simulink model "hearingAid_System_v1"  (R2026a)
settings: Solver=VariableStepAuto
undefined symbols (not defined in the file): bHigh, bLow, bMid, dspblkCoreblockFVToolHelper, gcbh
libraries: audiodynamicrange x2, dspstat3 x2, dspmathops x2, audiofilters x2, dspvision x1, dspsnks4 x1, dspsigops x1
settings Model: Creator=admin  LastModifiedBy=shami

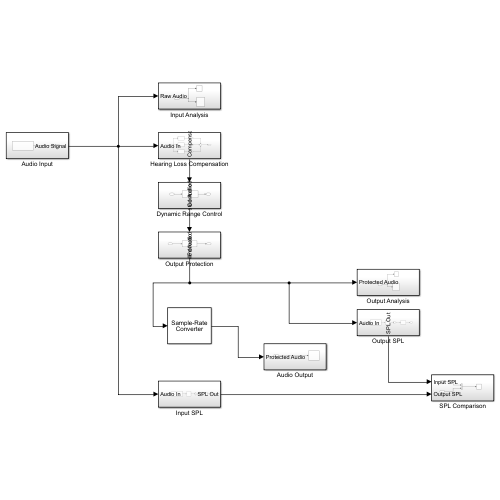
[thumbnail: Simulink's stored preview of the top-level diagram]
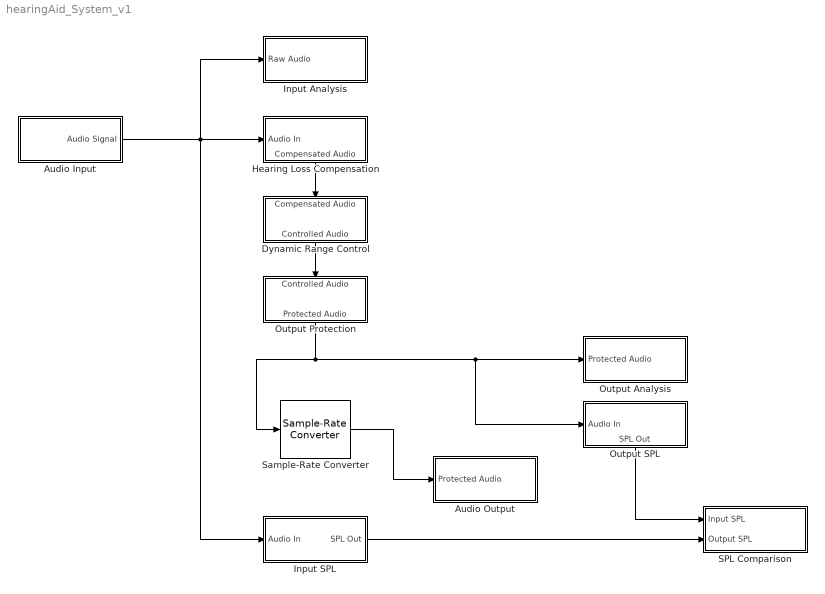
== system hearingAid_System_v1 ==
  Audio Input : Subsystem
  Audio Output : Subsystem
  Dynamic Range Control : Subsystem  Description=|
      | Controls the amplitude dynamics of the compensated signal using compression followed by 
      | peak limiting. The compressor reduces excessive level variations, while the limiter prevents 
      | high-amplitude transients from exceeding the selected threshold.
      settings: PortSchema="{\"entries\":[{\"content\":{\"sides\":[{\"content\":{},\"type\":\"ConnectorPlacement.EquallySpacedRectSide\",\"uuid\":\"9fa1bc4c-7734-4da4-8790-dcaf3a5a96d7\"},{\"content\":{\"side\":\"RIGHT\"},\"type\":\"ConnectorPlacement.EquallySpacedRectSide\",\"uuid\":\"a0bb4f64-da4e-44f2-8384-5606d89d98dc\"},{\"content\":{\"connectorIds\":[\"In1\"],\"side\":\"TOP\"},\"type\":\"ConnectorPlacement.EquallySpacedRectSide\",\"uuid\":\"07e91a7b-911d-4066-a5e2-6f66f183605b\"},{\"content\":{\"connectorIds\":[\"Out1\"],\"side\":\"BOTTOM\"},\"type\":\"ConnectorPlacement.EquallySpacedRectSide\",\"uuid\":\"dc75b34e-663d-4060-af1f-fa3536e55f2f\"}]},\"type\":\"ConnectorPlacement.EquallySpacedConnector\",\"uuid\":\"5366c7c7-2506-4129-8805-fe24e186531d\"}],\"packageUris\":[\"http://schema.mathworks.com/mf0/Connector/R2020b\"],\"version\":\"1.0\"}"
  Hearing Loss Compensation : Subsystem  Description=|
      | Separates the input audio into low-, mid-, and high-frequency bands using matched-delay 
      | FIR filters. Independent prescription gains are applied to each band and the signals are 
      | recombined to produce the compensated audio signal.
      settings: PortSchema="{\"entries\":[{\"content\":{\"sides\":[{\"content\":{\"connectorIds\":[\"In1\"]},\"type\":\"ConnectorPlacement.EquallySpacedRectSide\",\"uuid\":\"9fa1bc4c-7734-4da4-8790-dcaf3a5a96d7\"},{\"content\":{\"side\":\"RIGHT\"},\"type\":\"ConnectorPlacement.EquallySpacedRectSide\",\"uuid\":\"a0bb4f64-da4e-44f2-8384-5606d89d98dc\"},{\"content\":{\"side\":\"TOP\"},\"type\":\"ConnectorPlacement.EquallySpacedRectSide\",\"uuid\":\"07e91a7b-911d-4066-a5e2-6f66f183605b\"},{\"content\":{\"connectorIds\":[\"Out1\"],\"side\":\"BOTTOM\"},\"type\":\"ConnectorPlacement.EquallySpacedRectSide\",\"uuid\":\"08ca0ef5-9875-4344-8c5b-4fbce4711590\"}]},\"type\":\"ConnectorPlacement.EquallySpacedConnector\",\"uuid\":\"5366c7c7-2506-4129-8805-fe24e186531d\"}],\"packageUris\":[\"http://schema.mathworks.com/mf0/Connector/R2020b\"],\"version\":\"1.0\"}"
  Input Analysis : Subsystem  Description=|
      | Analyzes the incoming audio signal in the time and frequency domains before hearing-aid 
      | processing. The subsystem provides waveform and spectral views of the original signal for 
      | comparison with the processed output.
  Input SPL : Subsystem  Description=|
      | Estimates the A-weighted sound pressure level of the input audio using frequency weighting 
      | and moving RMS measurement. The resulting level is provided for real-time monitoring and 
      | comparison with the processed signal.
  Output Analysis : Subsystem  Description=|
      | Monitors the processed audio in the time and frequency domains after dynamic range control. 
      | The waveform and spectrum provide direct evidence of changes introduced by the hearing-aid 
      | processing chain.
  Output Protection : Subsystem  Description=|
      | Protects the compensated audio from excessive amplitude peaks before playback. The 
      | subsystem applies final peak-level control to prevent clipping and maintain a controlled 
      | signal level for the downstream audio output stage.
      settings: PortSchema="{\"entries\":[{\"content\":{\"sides\":[{\"content\":{},\"type\":\"ConnectorPlacement.EquallySpacedRectSide\",\"uuid\":\"9fa1bc4c-7734-4da4-8790-dcaf3a5a96d7\"},{\"content\":{\"side\":\"RIGHT\"},\"type\":\"ConnectorPlacement.EquallySpacedRectSide\",\"uuid\":\"a0bb4f64-da4e-44f2-8384-5606d89d98dc\"},{\"content\":{\"connectorIds\":[\"In1\"],\"side\":\"TOP\"},\"type\":\"ConnectorPlacement.EquallySpacedRectSide\",\"uuid\":\"07e91a7b-911d-4066-a5e2-6f66f183605b\"},{\"content\":{\"connectorIds\":[\"Out1\"],\"side\":\"BOTTOM\"},\"type\":\"ConnectorPlacement.EquallySpacedRectSide\",\"uuid\":\"e48d2dd4-e7e7-47b9-be68-aa31b977a762\"}]},\"type\":\"ConnectorPlacement.EquallySpacedConnector\",\"uuid\":\"5366c7c7-2506-4129-8805-fe24e186531d\"}],\"packageUris\":[\"http://schema.mathworks.com/mf0/Connector/R2020b\"],\"version\":\"1.0\"}"
  Output SPL : Subsystem  Description=|
      | Measures the A-weighted sound pressure level after hearing-aid processing using the same 
      | measurement chain as the input stage, enabling a consistent input-versus-output level 
      | comparison.
      settings: PortSchema="{\"entries\":[{\"content\":{\"sides\":[{\"content\":{\"connectorIds\":[\"In1\"]},\"type\":\"ConnectorPlacement.EquallySpacedRectSide\",\"uuid\":\"9fa1bc4c-7734-4da4-8790-dcaf3a5a96d7\"},{\"content\":{\"side\":\"RIGHT\"},\"type\":\"ConnectorPlacement.EquallySpacedRectSide\",\"uuid\":\"a0bb4f64-da4e-44f2-8384-5606d89d98dc\"},{\"content\":{\"side\":\"TOP\"},\"type\":\"ConnectorPlacement.EquallySpacedRectSide\",\"uuid\":\"07e91a7b-911d-4066-a5e2-6f66f183605b\"},{\"content\":{\"connectorIds\":[\"Out1\"],\"side\":\"BOTTOM\"},\"type\":\"ConnectorPlacement.EquallySpacedRectSide\",\"uuid\":\"6873dc33-1ba5-4860-bfcc-e1687ab0e849\"}]},\"type\":\"ConnectorPlacement.EquallySpacedConnector\",\"uuid\":\"5366c7c7-2506-4129-8805-fe24e186531d\"}],\"packageUris\":[\"http://schema.mathworks.com/mf0/Connector/R2020b\"],\"version\":\"1.0\"}"
  SPL Comparison : Subsystem  Description=|
      | Compares the measured input and output sound pressure levels on a common time axis to 
      | visualize the level changes produced by the hearing-aid processing system.
  Sample-Rate Converter : dspsigops/Sample-Rate Converter  InputSampleRate=16000  OutputSampleRate=48000  OutputRateTolerance=0  Bandwidth=7500  StopbandAttenuation=80  AllowArbitraryInputLength=off  SimulateUsing=Interpreted execution
      settings: LibrarySourceBlock=|
      | dspmlti4/Sample-Rate
      | Converter
  wires:
  Sample-Rate Converter/1 -> Audio Output/1(Protected Audio)
  Dynamic Range Control/1(Controlled Audio) -> Output Protection/1(Controlled Audio)
  Output SPL/1(SPL Out) -> SPL Comparison/1(Input SPL)
  Hearing Loss Compensation/1(Compensated Audio) -> Dynamic Range Control/1(Compensated Audio)
  Audio Input/1(Audio Signal) -> Input SPL/1(Audio In), Input Analysis/1(Raw Audio), Hearing Loss Compensation/1(Audio In)
  Output Protection/1(Protected Audio) -> Output Analysis/1(Protected Audio), Output SPL/1(Audio In), Sample-Rate Converter/1
  Input SPL/1(SPL Out) -> SPL Comparison/2(Output SPL)

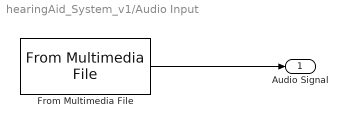
== system hearingAid_System_v1/Audio Input ==
  From Multimedia File : dspvision/From Multimedia File  inputFilename=E:\SS Project\Simulink-Hearing-Aid\Data\datasets\TIMIT\TRAIN\DR1\FCJF0\SA1.WAV  readRange=[1 Inf]  loop=on  numPlays=1  outputStreams=Audio only  videoDataType=single  audioDataType=double  inheritSampleTime=on  userDefinedSampleTime=1/30  noAudioOutput=off  isIntensityVideo=off  fourcc=RGB  colorVideoFormat=Separate color signals  outputEOF=off  dataOrg=Column-major  audioFrameSize=1024  computeAudioFrameSize=off  outSamplingMode=Sample based
      settings: LibrarySourceBlock=audiosources/From Multimedia File
  Audio Signal : Outport
  wires:
  From Multimedia File/1 -> Audio Signal/1

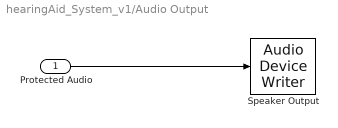
== system hearingAid_System_v1/Audio Output ==
  Protected Audio : Inport
  Speaker Output : dspsnks4/Audio Device Writer  Driver=DirectSound  Device=Default  InheritSampleRate=off  SampleRate=44100  BitDepth=16-bit integer  BufferSize=4096  NumBuffers=10  DefaultOutputChannelMapping=on  OutputChannelMapping=1:2  OutputNumUnderrunSamples=off  DriverIdx=1  DeviceWarnFlag=''
  wires:
  Protected Audio/1 -> Speaker Output/1

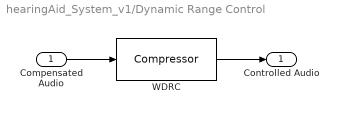
== system hearingAid_System_v1/Dynamic Range Control ==
  Compensated Audio : Inport
  WDRC : audiodynamicrange/Compressor  ThresholdPort=off  Threshold=-10.0  RatioPort=off  Ratio=5.0  KneeWidthPort=off  KneeWidth=0.0  AttackTimePort=off  AttackTime=0.05  ReleaseTimePort=off  ReleaseTime=0.2  MakeUpGainMode=Property  MakeUpGain=0.0  InheritSampleRate=off  SampleRate=16000  outputGain=off  EnableSidechain=off  SimulateUsing=Interpreted execution
  Controlled Audio : Outport
  wires:
  Compensated Audio/1 -> WDRC/1
  WDRC/1 -> Controlled Audio/1

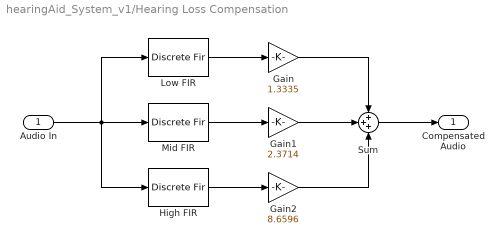
== system hearingAid_System_v1/Hearing Loss Compensation ==
  Audio In : Inport
  Gain : Gain  Gain=1.3335
  Gain1 : Gain  Gain=2.3714
  Gain2 : Gain  Gain=8.6596
  High FIR : DiscreteFir  LoadFcn=dspblkCoreblockFVToolHelper(gcbh,'load');  Coefficients=bHigh  InputProcessing=Columns as channels (frame based)
      settings: CopyFcn=dspblkCoreblockFVToolHelper(gcbh,'copy');  DeleteFcn=dspblkCoreblockFVToolHelper(gcbh,'close');  ModelCloseFcn=dspblkCoreblockFVToolHelper(gcbh,'close');  PreSaveFcn=dspblkCoreblockFVToolHelper(gcbh,'presave');  PostSaveFcn=dspblkCoreblockFVToolHelper(gcbh,'postsave');  CloseFcn=dspblkCoreblockFVToolHelper(gcbh,'close');
  Low FIR : DiscreteFir  LoadFcn=dspblkCoreblockFVToolHelper(gcbh,'load');  Coefficients=bLow  InputProcessing=Columns as channels (frame based)
      settings: CopyFcn=dspblkCoreblockFVToolHelper(gcbh,'copy');  DeleteFcn=dspblkCoreblockFVToolHelper(gcbh,'close');  ModelCloseFcn=dspblkCoreblockFVToolHelper(gcbh,'close');  PreSaveFcn=dspblkCoreblockFVToolHelper(gcbh,'presave');  PostSaveFcn=dspblkCoreblockFVToolHelper(gcbh,'postsave');  CloseFcn=dspblkCoreblockFVToolHelper(gcbh,'close');
  Mid FIR : DiscreteFir  LoadFcn=dspblkCoreblockFVToolHelper(gcbh,'load');  Coefficients=bMid  InputProcessing=Columns as channels (frame based)
      settings: CopyFcn=dspblkCoreblockFVToolHelper(gcbh,'copy');  DeleteFcn=dspblkCoreblockFVToolHelper(gcbh,'close');  ModelCloseFcn=dspblkCoreblockFVToolHelper(gcbh,'close');  PreSaveFcn=dspblkCoreblockFVToolHelper(gcbh,'presave');  PostSaveFcn=dspblkCoreblockFVToolHelper(gcbh,'postsave');  CloseFcn=dspblkCoreblockFVToolHelper(gcbh,'close');
  Sum : Sum  Inputs=+++
  Compensated Audio : Outport
  wires:
  Audio In/1 -> Low FIR/1, High FIR/1, Mid FIR/1
  Low FIR/1 -> Gain/1
  Mid FIR/1 -> Gain1/1
  High FIR/1 -> Gain2/1
  Gain/1 -> Sum/1
  Gain1/1 -> Sum/2
  Gain2/1 -> Sum/3
  Sum/1 -> Compensated Audio/1

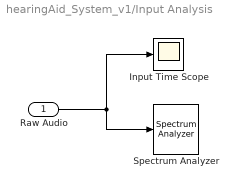
== system hearingAid_System_v1/Input Analysis ==
  Raw Audio : Inport
  Input Time Scope : Scope
      settings: TimeSpan=10  TimeUnits=Metric (based on Time Span)  YLabel=Amplitude
  Spectrum Analyzer : SpectrumAnalyzer  WindowPosition=[219.000000,126.000000,800.000000,500.000000,]  ScopeFrameLocation=window  SampleRate=44.1e3  PlotAsTwoSidedSpectrum=off  FrequencyScale=Log  WindowInvariantSamplesPerUpdate=on  FrequencySpan=Start and stop frequencies  StartFrequency=0  StopFrequency=8000  YLimits=[-99.7211 -44.223]  ShowLegend=on  SelectedToolstripTab=spectrumAnalyzerToolstrip.estimationTab
  wires:
  Raw Audio/1 -> Spectrum Analyzer/1, Input Time Scope/1

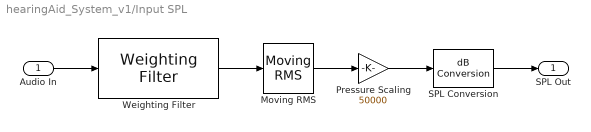
== system hearingAid_System_v1/Input SPL ==
  Audio In : Inport
  Moving RMS : dspstat3/Moving RMS  Method=Sliding window  ForgettingFactorPort=off  SpecifyWindowLength=on  WindowLength=1024  OverlapLength=0  AllowArbitraryInputLength=off  ForgettingFactor=0.9  SimulateUsing=Interpreted execution
  Pressure Scaling : Gain  Gain=50000
  SPL Conversion : dspmathops/dB Conversion  dBtype=dB  intype=Amplitude  R=1  fuzz=off
  Weighting Filter : audiofilters/Weighting Filter  Method=A-weighting  InheritSampleRate=on  SampleRate=44100  SimulateUsing=Interpreted execution  WorkspaceVariableName=myFilt  OverwriteExportVariable=on  MaskClassType=No mask
  SPL Out : Outport
  wires:
  Audio In/1 -> Weighting Filter/1
  Weighting Filter/1 -> Moving RMS/1
  Moving RMS/1 -> Pressure Scaling/1
  Pressure Scaling/1 -> SPL Conversion/1
  SPL Conversion/1 -> SPL Out/1

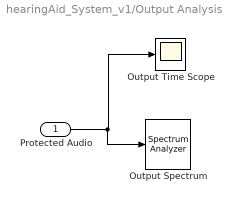
== system hearingAid_System_v1/Output Analysis ==
  Protected Audio : Inport
  Output Spectrum : SpectrumAnalyzer  WindowPosition=[894.000000,-152.000000,800.000000,500.000000,]  ScopeFrameLocation=window  SampleRate=44.1e3  PlotAsTwoSidedSpectrum=off  FrequencyScale=Log  WindowInvariantSamplesPerUpdate=on  FrequencySpan=Start and stop frequencies  StartFrequency=0  StopFrequency=8000  YLimits=[-85.3104 -37.6205]  SelectedToolstripTab=spectrumAnalyzerToolstrip.estimationTab
  Output Time Scope : Scope
      settings: TimeSpan=10  TimeUnits=Metric (based on Time Span)  ActiveDisplayYMinimum=-0.30126545077203903  ActiveDisplayYMaximum=0.37204010677583255  YLabel=Amplitude
  wires:
  Protected Audio/1 -> Output Spectrum/1, Output Time Scope/1

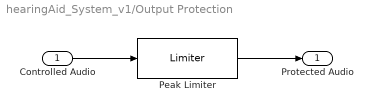
== system hearingAid_System_v1/Output Protection ==
  Controlled Audio : Inport
  Peak Limiter : audiodynamicrange/Limiter  ThresholdPort=off  Threshold=-10.0  KneeWidthPort=off  KneeWidth=0.0  AttackTimePort=off  AttackTime=0.0  ReleaseTimePort=off  ReleaseTime=0.2  MakeUpGainMode=Property  MakeUpGain=0.0  InheritSampleRate=off  SampleRate=16000  outputGain=off  EnableSidechain=off  SimulateUsing=Interpreted execution
  Protected Audio : Outport
  wires:
  Controlled Audio/1 -> Peak Limiter/1
  Peak Limiter/1 -> Protected Audio/1

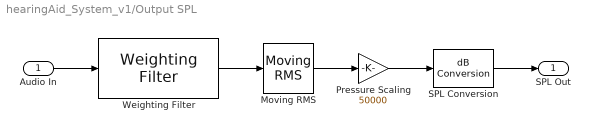
== system hearingAid_System_v1/Output SPL ==
  Audio In : Inport
  Moving RMS : dspstat3/Moving RMS  Method=Sliding window  ForgettingFactorPort=off  SpecifyWindowLength=on  WindowLength=1024  OverlapLength=0  AllowArbitraryInputLength=off  ForgettingFactor=0.9  SimulateUsing=Interpreted execution
  Pressure Scaling : Gain  Gain=50000
  SPL Conversion : dspmathops/dB Conversion  dBtype=dB  intype=Amplitude  R=1  fuzz=off
  Weighting Filter : audiofilters/Weighting Filter  Method=A-weighting  InheritSampleRate=on  SampleRate=44100  SimulateUsing=Interpreted execution  WorkspaceVariableName=myFilt  OverwriteExportVariable=on  MaskClassType=No mask
  SPL Out : Outport
  wires:
  Audio In/1 -> Weighting Filter/1
  Weighting Filter/1 -> Moving RMS/1
  Moving RMS/1 -> Pressure Scaling/1
  Pressure Scaling/1 -> SPL Conversion/1
  SPL Conversion/1 -> SPL Out/1

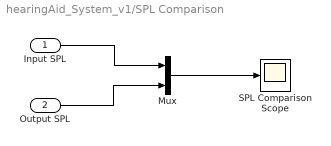
== system hearingAid_System_v1/SPL Comparison ==
  Input SPL : Inport
  Output SPL : Inport  Port=2
  Mux : Mux  Inputs=2
  SPL Comparison Scope : Scope
      settings: TimeUnits=Metric (based on Time Span)  ActiveDisplayYMinimum=-3512.1611498709003  ActiveDisplayYMaximum=473.27708174153668  YLabel=Amplitude  DataLoggingVariableName=ScopeData2
  wires:
  Input SPL/1 -> Mux/1
  Output SPL/1 -> Mux/2
  Mux/1 -> SPL Comparison Scope/1
